simulink model "takeoff23b"  (R2025b)
settings: Solver=ode4  StartTime=0.0  StopTime=150  FixedStep=0.001  RelTol=1e-3
values from neighbouring files (symbols this model uses):
  a0 = 340.294    [basedata.m]    (also in basedata.mat; landing_init.m; landing_plan.mat; landingplan.mat)
  b_ref = 2.0    (= 2)    [basedata.m]    (also in basedata.mat; landing_init.m; landing_plan.mat; landingplan.mat)
  c_gear = [0.8e4, 1.4e4, 1.4e4]    [basedata.m]    (also in basedata.mat = [8000 14000 14000]; landing_init.m; landing_plan.mat = [8000 14000 14000]; landingplan.mat = [8000 14000 14000])
  c_lat = [1.4e4, 2.2e4, 2.2e4]    [basedata.m]    (also in basedata.mat = [14000 22000 22000]; landing_init.m; landing_plan.mat = [14000 22000 22000]; landingplan.mat = [14000 22000 22000])
  c_ref = 0.9    [basedata.m]    (also in basedata.mat; landing_init.m; landing_plan.mat; landingplan.mat)
  c_roll = [0.020, 0.018, 0.018]    [basedata.m]    (also in basedata.mat = [0.02 0.018 0.018]; landing_init.m; landing_plan.mat = [0.02 0.018 0.018]; landingplan.mat = [0.02 0.018 0.018])
  CD0 = 0.045    [basedata.m]    (also in basedata.mat; canshujisuan.m; landing_init.m; landing_plan.mat)
  CL0 = 0.083    [basedata.m]    (also in basedata.mat; landing_init.m; landing_plan.mat; landing_trajectory.m)
  CLa = 3.80    (= 3.8)    [basedata.m]    (also in basedata.mat; canshujisuan.m = 2.5; landing_init.m; landing_plan.mat)
  Clb = -0.08    [basedata.m]    (also in basedata.mat; landing_init.m; landing_plan.mat; landingplan.mat)
  Clda = -0.20    (= -0.2)    [basedata.m]    (also in basedata.mat; landing_init.m; landing_plan.mat; landingplan.mat)
  CLde = 0.28    [basedata.m]    (also in basedata.mat; landing_init.m; landing_plan.mat; landingplan.mat)
  Clp = -0.70    (= -0.7)    [basedata.m]    (also in basedata.mat; landing_init.m; landing_plan.mat; landingplan.mat)
  CLq = 4.50    (= 4.5)    [basedata.m]    (also in basedata.mat; canshujisuan.m = 3; landing_init.m; landing_plan.mat)
  Clr = 0.08    [basedata.m]    (also in basedata.mat; landing_init.m; landing_plan.mat; landingplan.mat)
  Cm0 = 0.060    (= 0.06)    [basedata.m]    (also in basedata.mat; landing_init.m; landing_plan.mat; landingplan.mat)
  Cma = -0.80    (= -0.8)    [basedata.m]    (also in basedata.mat; landing_init.m; landing_plan.mat; landingplan.mat)
  Cmde = -0.90    (= -0.9)    [basedata.m]    (also in basedata.mat; landing_init.m; landing_plan.mat; landingplan.mat)
  Cmq = -18.0    (= -18)    [basedata.m]    (also in basedata.mat; landing_init.m; landing_plan.mat; landingplan.mat)
  Cnb = 0.25    [basedata.m]    (also in basedata.mat; landing_init.m; landing_plan.mat; landingplan.mat)
  Cndr = -0.15    [basedata.m]    (also in basedata.mat; landing_init.m; landing_plan.mat; landingplan.mat)
  Cnp = -0.04    [basedata.m]    (also in basedata.mat; landing_init.m; landing_plan.mat; landingplan.mat)
  Cnr = -0.45    [basedata.m]    (also in basedata.mat; landing_init.m; landing_plan.mat; landingplan.mat)
  CSb = -0.70    (= -0.7)    [basedata.m]    (also in basedata.mat; landing_init.m; landing_plan.mat; landingplan.mat)
  CSdr = 0.18    [basedata.m]    (also in basedata.mat; landing_init.m; landing_plan.mat; landingplan.mat)
  CSr = 0.12    [basedata.m]    (also in basedata.mat; landing_init.m; landing_plan.mat; landingplan.mat)
  D = 0.5 * rho0 * V^2 * S_ref * CD_current    [canshujisuan.m]
  D0 = 1400    [basedata.m]    (also in basedata.mat; landing.m; landing_init.m; landing_plan.mat)
  da_max = 25    [basedata.m]    (also in basedata.mat; landing_init.m; landing_plan.mat; landingplan.mat)
  da_min = -da_max    (= -25)    [basedata.m]    (also in basedata.mat; landing_init.m; landing_plan.mat; landingplan.mat)
  de_max = 25    [basedata.m]    (also in basedata.mat; landing_init.m; landing_plan.mat; landingplan.mat)
  de_min = -de_max    (= -25)    [basedata.m]    (also in basedata.mat; landing_init.m; landing_plan.mat; landingplan.mat)
  DH = pi / 180    (= 0.0174532925199)    [basedata.m]    (also in basedata.mat; landing_init.m; landing_plan.mat; landingplan.mat)
  dr_max = 25    [basedata.m]    (also in basedata.mat; landing_init.m; landing_plan.mat; landingplan.mat)
  dr_min = -dr_max    (= -25)    [basedata.m]    (also in basedata.mat; landing_init.m; landing_plan.mat; landingplan.mat)
  g = 9.80665    [basedata.m]    (also in basedata.mat; canshujisuan.m; landing_init.m; landing_plan.mat)
  gamma1 = -0.125844364415    [basedata.mat]    (also in landing_trajectory.m = asin((T_idle - D_app) / (m*g)); landingplan.mat)
  gamma2 = -0.0261780104712    [basedata.mat]    (also in landing_trajectory.m; landingplan.mat)
  ground_z = 0.0    (= 0)    [basedata.m]    (also in basedata.mat; landing_init.m; landing_plan.mat; landingplan.mat)
  HD = 180 / pi    (= 57.2957795131)    [basedata.m]    (also in basedata.mat; landing_init.m; landing_plan.mat; landingplan.mat)
  I = [ Ixx, -Ixy, -Ixz ... (first row only)    [basedata.m]    (also in basedata.mat = [120  0  0; 0  480  0; 0  0  520]; landing_init.m; landing_plan.mat = [120  0  0; 0  480  0; 0  0  520]; landingplan.mat = [120  0  0; 0  480  0; 0  0  520])
  K = 0.12    [basedata.m]    (also in basedata.mat; canshujisuan.m = 0.08; landing_init.m; landing_plan.mat)
  K_alpha = 7.5375    [basedata.mat]    (also in control_design.m = (((wd_pitch^2)-a24))/(2*kesi_pitch*wd_pitch); control_design.mat; controller.m = 5; landingplan.mat)
  k_gear = [1.0e5, 3.0e5, 3.0e5]    [basedata.m]    (also in basedata.mat = [100000 300000 300000]; landing_init.m; landing_plan.mat = [100000 300000 300000]; landingplan.mat = [100000 300000 300000])
  Kn_pitch = -0.120095403309    [basedata.mat]    (also in control_design.m = -(2.2*g*(wd_pitch)^2)/(Tr*(((wd_pitch)^2)-a24)*V_control*a34; control_design.mat; controller.m = (2.2*wd^2*g)/(Tr*(wd^2-a24)*V_test*a34); landingplan.mat)
  Kw_pitch = -0.483749055178    [basedata.mat]    (also in control_design.m = -2*kesi_pitch*wd_pitch/a25; control_design.mat; controller.m = -(2*zeta*wd) / a25; landingplan.mat)
  m = 600.0    (= 600)    [basedata.m]    (also in basedata.mat; canshujisuan.m; landing_init.m; landing_plan.mat)
  mu_brake = [0.0, 0.55, 0.55]    [basedata.m]    (also in basedata.mat = [0 0.55 0.55]; landing_init.m; landing_plan.mat = [0 0.55 0.55]; landingplan.mat = [0 0.55 0.55])
  phi0 = 0.0    (= 0)    [landing.m]    (also in landing_init.m; landing_init.mat; landing_plan.mat; landingplan.mat)
  psi0 = 0.0    (= 0)    [landing.m]    (also in landing_init.m; landing_init.mat; landing_plan.mat; landingplan.mat)
  r_left_b = r_gear_b(:,2)    [basedata.m]    (also in basedata.mat = [-0.333333333333 -0.8 0.65]; landing_init.m; landing_plan.mat = [-0.333333333333 -0.8 0.65]; landingplan.mat = [-0.333333333333 -0.8 0.65])
  r_nose_b = r_gear_b(:,1)    [basedata.m]    (also in basedata.mat = [2 0 0.65]; landing_init.m; landing_plan.mat = [2 0 0.65]; landingplan.mat = [2 0 0.65])
  r_right_b = r_gear_b(:,3)    [basedata.m]    (also in basedata.mat = [-0.333333333333 0.8 0.65]; landing_init.m; landing_plan.mat = [-0.333333333333 0.8 0.65]; landingplan.mat = [-0.333333333333 0.8 0.65])
  rho0 = 1.225    [basedata.m]    (also in basedata.mat; canshujisuan.m; landing_init.m; landing_plan.mat)
  S_ref = 1.2    [basedata.m]    (also in basedata.mat; canshujisuan.m; landing_init.m; landing_plan.mat)
  theta0 = 0.0    (= 0)    [landing.m]    (also in landing_init.m; landing_init.mat = 0.0523598775598; landing_plan.mat = 0.0523560209424; landingplan.mat)
  u0_b = 128.0    (= 128)    [landing.m]    (also in landing_init.m; landing_init.mat = 100; landing_plan.mat; landingplan.mat)
  v0_b = 0.0    (= 0)    [landing.m]    (also in landing_init.m; landing_init.mat; landing_plan.mat; landingplan.mat)
  v_eps = 0.20    (= 0.2)    [basedata.m]    (also in basedata.mat; landing_init.m; landing_plan.mat; landingplan.mat)
  V_min = 3    [landing.m]    (also in landing_init.m; landing_plan.mat; landingplan.mat; plan.m = 1)
  w0_b = 0.0    (= 0)    [landing.m]    (also in landing_init.m; landing_init.mat; landing_plan.mat; landingplan.mat)
  wheel_radius = 0.18    [basedata.m]    (also in basedata.mat; landing_init.m; landing_plan.mat; landingplan.mat)
  WOW_on = 0.000    (= 0)    [basedata.m]    (also in basedata.mat; landing_init.m; landing_plan.mat; landingplan.mat)
  Xg0 = -12000.0    (= -12000)    [landing.m]    (also in landing_init.m; landing_init.mat = -8000; landing_plan.mat; landingplan.mat)
  Yg0 = 0.0    (= 0)    [landing.m]    (also in landing_init.m; landing_init.mat; landing_plan.mat; landingplan.mat)
  Zg0 = ground_z - wheel_radius - r_gear_b(3,1) + static_deflection    [basedata.m]    (also in basedata.mat = -0.8215943; landing.m = -1000; landing_init.m = -1000; landing_init.mat = -350)
undefined symbols (not defined in the file or in its folder): I_xz, I_yz, Ix_Iy, Iy_Iz, Iz_Ix
libraries: simulink x58, matrix_library x19
(part 4 of 4)

== matlab function takeoff23b/6DOF-MODEL/动力学/Subsystem3/MATLAB Function ==
  data: phi input; R_bg output; theta input; psi input
function R_bg = ground2body(phi, theta, psi)
T1 = [cos(psi), sin(psi), 0;
     -sin(psi), cos(psi), 0;
      0, 0, 1];
T2 = [cos(theta), 0, -sin(theta);
       0, 1, 0;
      sin(theta), 0, cos(theta)];
T3 = [1, 0, 0;
      0, cos(phi), sin(phi);
      0, -sin(phi), cos(phi)];
R_bg = T3 * T2 * T1;

== matlab function takeoff23b/6DOF-MODEL/动力学/dynamics EQ/MATLAB Function ==
  data: alpha input; R_bwind output; beta input
function R_bwind = wind2body(alpha, beta)
T1 = [cos(alpha), 0, sin(alpha);
       0, 1, 0;
       -sin(alpha), 0, cos(alpha)];
T2 = [cos(beta), sin(beta), 0;
       -sin(beta), cos(beta), 0;
       0, 0, 1];
R_wind_b = T2*T1;
R_bwind = R_wind_b';

== matlab function takeoff23b/controller1/4_Power&V_Ctrl/MATLAB Function ==
  data: Vel_g input; dv_err output; axyz input
function dv_err = dv_cal(Vel_g,axyz)
%#codegen

% k_theta = Att_g(1)*pi/180;
% psi = Att_g(2)*pi/180;
% gama = Att_g(3)*pi/180;
% 
% Cg_b = Mx(gama)*Mz(k_theta)*My(psi);
% Cb_g = Cg_b';
vx = Vel_g(1);
vy = Vel_g(2);
vz = Vel_g(3);

ax = axyz(1);
ay = axyz(2);
az = axyz(3);

dv_err = (vx*ax + vy*ay + vz*az)/sqrt(vx^2 + vy^2 + vz^2);
% dv_err = (vx*ax + vz*az)/sqrt(vx^2 + vz^2);
if isnan(dv_err) == 1 
    dv_err = 0;
end

== matlab function takeoff23b/6DOF-MODEL/动力学/dynamics EQ/MATLAB Function1 ==
  data: phi input; R_bg output; theta input; psi input
function R_bg = ground2body(phi, theta, psi)
T1 = [cos(psi), sin(psi), 0;
     -sin(psi), cos(psi), 0;
      0, 0, 1];
T2 = [cos(theta), 0, -sin(theta);
       0, 1, 0;
      sin(theta), 0, cos(theta)];
T3 = [1, 0, 0;
      0, cos(phi), sin(phi);
      0, -sin(phi), cos(phi)];
R_bg = T3 * T2 * T1;

== matlab function takeoff23b/6DOF-MODEL/动力学/height/MATLAB Function ==
  data: phi input; R_bg output; theta input; psi input
function R_bg = ground2body(phi, theta, psi)
T1 = [cos(psi), sin(psi), 0;
     -sin(psi), cos(psi), 0;
      0, 0, 1];
T2 = [cos(theta), 0, -sin(theta);
       0, 1, 0;
      sin(theta), 0, cos(theta)];
T3 = [1, 0, 0;
      0, cos(phi), sin(phi);
      0, -sin(phi), cos(phi)];
R_bg = T3 * T2 * T1;

== matlab function takeoff23b/6DOF-MODEL/动力学/rotation EQ/MATLAB Function1 ==
  data: w input; wB_X output
function wB_X = wB_X(w) 
p = w(1);
q = w(2);
r = w(3);
wB_X = [0, -r,  q;...
        r,  0, -p;...
       -q,  p,  0];

== matlab function takeoff23b/6DOF-MODEL/动力学/起落架模型/MATLAB Function ==
  data: phi input; R_bg output; theta input; psi input
function R_bg = ground2body(phi, theta, psi)
T1 = [cos(psi), sin(psi), 0;
     -sin(psi), cos(psi), 0;
      0, 0, 1];
T2 = [cos(theta), 0, -sin(theta);
       0, 1, 0;
      sin(theta), 0, cos(theta)];
T3 = [1, 0, 0;
      0, cos(phi), sin(phi);
      0, -sin(phi), cos(phi)];
R_bg = T3 * T2 * T1;

== matlab function takeoff23b/6DOF-MODEL/动力学/起落架模型/侧向力/Subsystem/MATLAB Function ==
  data: phi input; R_bg output; theta input; psi input
function R_bg = ground2body(phi, theta, psi)
T1 = [cos(psi), sin(psi), 0;
     -sin(psi), cos(psi), 0;
      0, 0, 1];
T2 = [cos(theta), 0, -sin(theta);
       0, 1, 0;
      sin(theta), 0, cos(theta)];
T3 = [1, 0, 0;
      0, cos(phi), sin(phi);
      0, -sin(phi), cos(phi)];
R_bg = T3 * T2 * T1;

== matlab function takeoff23b/6DOF-MODEL/动力学/起落架模型/侧向力/Subsystem/主轮侧向方向向量 ==
  data: Cbg input; eg_lat output; eb_lat input
function eg_lat = project_main_lat(Cbg, eb_lat)

e_z = [0; 0; 1];              % 前-右-下坐标系：Z 轴向下
P_g = eye(3) - e_z*e_z.';     % 投影到地面水平面

eg_lat = P_g * Cbg * eb_lat;

n = norm(eg_lat);
if n > 1e-8
    eg_lat = eg_lat / n;
else
    eg_lat = [0; 1; 0];       % 默认地面右向
end

== matlab function takeoff23b/6DOF-MODEL/动力学/起落架模型/侧向力/Subsystem/前轮侧向向量 ==
  data: Cbg input; eg_lat output; eb_lat input
function eg_lat = project_lat(Cbg, eb_lat)

e_z = [0; 0; 1];              % 前-右-下坐标系：Z 轴向下
P_g = eye(3) - e_z*e_z.';     % 投影到地面水平面

eg_lat = P_g * Cbg * eb_lat;

n = norm(eg_lat);
if n > 1e-8
    eg_lat = eg_lat / n;
else
    eg_lat = [0; 1; 0];       % 默认地面右向
end

== matlab function takeoff23b/6DOF-MODEL/动力学/起落架模型/MATLAB Function1 ==
  data: phi input; R_bg output; theta input; psi input
function R_bg = ground2body(phi, theta, psi)
T1 = [cos(psi), sin(psi), 0;
     -sin(psi), cos(psi), 0;
      0, 0, 1];
T2 = [cos(theta), 0, -sin(theta);
       0, 1, 0;
      sin(theta), 0, cos(theta)];
T3 = [1, 0, 0;
      0, cos(phi), sin(phi);
      0, -sin(phi), cos(phi)];
R_bg = T3 * T2 * T1;

== matlab function takeoff23b/6DOF-MODEL/动力学/起落架模型/三轮在地系下的力/摩擦圆限幅/前轮摩擦圆限幅 ==
  data: N input; F_long_out output; F_long input; F_lat input; F_lat_out output
function [F_long_out,F_lat_out]=Dround_saturation_nose(N,F_long,F_lat)
mu=0.65;
F_ALL=sqrt((F_long)^2+(F_lat)^2);
if(F_ALL<=mu*N)
    F_long_out=F_long;
    F_lat_out=F_lat;
else
    s=mu*N/F_ALL;
    F_long_out=s*F_long;
    F_lat_out=s*F_lat;
end

== matlab function takeoff23b/6DOF-MODEL/动力学/起落架模型/三轮在地系下的力/摩擦圆限幅/主轮摩擦圆限幅左 ==
  data: N input; F_long_out output; F_long input; F_lat input; F_lat_out output
function [F_long_out,F_lat_out]=Dround_saturation_main(N,F_long,F_lat)
mu=0.7;
F_ALL=sqrt((F_long)^2+(F_lat)^2);
if(F_ALL<=mu*N)
    F_long_out=F_long;
    F_lat_out=F_lat;
else
    s=mu*N/F_ALL;
    F_long_out=s*F_long;
    F_lat_out=s*F_lat;
end

== matlab function takeoff23b/6DOF-MODEL/动力学/起落架模型/三轮在地系下的力/摩擦圆限幅/主轮摩擦圆限幅右 ==
  data: N input; F_long_out output; F_long input; F_lat input; F_lat_out output
function [F_long_out,F_lat_out]=Dround_saturation_main(N,F_long,F_lat)
mu=0.7;
F_ALL=sqrt((F_long)^2+(F_lat)^2);
if(F_ALL<=mu*N)
    F_long_out=F_long;
    F_lat_out=F_lat;
else
    s=mu*N/F_ALL;
    F_long_out=s*F_long;
    F_lat_out=s*F_lat;
end

== matlab function takeoff23b/Guidance/3_空中制导/高度切换/MATLAB Function ==
  data: X_pos input; Hcmd output
function Hcmd = round_hcmd(X_pos)

X_B = -4048.3;
X_C = -3253.6;
X_R = -3044.2;
H_R = 8069.4;
R = 8000;

if X_pos >= X_B && X_pos <= X_C
    rad = R^2 - (X_pos - X_R)^2;
    Hcmd = H_R - sqrt(max(rad, 0));
else
    Hcmd = 0;
end

== matlab function takeoff23b/6DOF-MODEL/动力学/起落架模型/法向支反力/MATLAB Function ==
  data: phi input; R_bg output; theta input; psi input
function R_bg = ground2body(phi, theta, psi)
T1 = [cos(psi), sin(psi), 0;
     -sin(psi), cos(psi), 0;
      0, 0, 1];
T2 = [cos(theta), 0, -sin(theta);
       0, 1, 0;
      sin(theta), 0, cos(theta)];
T3 = [1, 0, 0;
      0, cos(phi), sin(phi);
      0, -sin(phi), cos(phi)];
R_bg = T3 * T2 * T1;

== matlab function takeoff23b/6DOF-MODEL/动力学/height/MATLAB Function1 ==
  data: phi input; R_bg output; theta input; psi input
function R_bg = ground2body(phi, theta, psi)
T1 = [cos(psi), sin(psi), 0;
     -sin(psi), cos(psi), 0;
      0, 0, 1];
T2 = [cos(theta), 0, -sin(theta);
       0, 1, 0;
      sin(theta), 0, cos(theta)];
T3 = [1, 0, 0;
      0, cos(phi), sin(phi);
      0, -sin(phi), cos(phi)];
R_bg = T3 * T2 * T1;

== stateflow chart takeoff23b/Flight Phase Manager/Phase Logic ==
  state Takeoff_Mode
    state Ground_Roll
      en: Flight_Phase = 1;
    state Rotation
      en: Flight_Phase = 2;
    state Liftoff
      en: Flight_Phase = 3;
    state Initial_Climb
      en: Flight_Phase = 4;
    state Climb_Complete
      en: Flight_Phase = 5;
    (default) -> Ground_Roll
    Ground_Roll -> Rotation : [reach_VR == true]
    Rotation -> Liftoff : [airborne == true]
    Liftoff -> Initial_Climb : [safe_climb == true]
    Initial_Climb -> Climb_Complete : [h_AGL  >= 800.0]
  state Landing_Mode
    state Glideslope_Capture
      en: Flight_Phase = 7;
    state Glideslope_Track
      en: Flight_Phase = 8;
    state Approach_Turn
      en: Flight_Phase = 6;
    state Roll_out
      en: Flight_Phase = 11;
    state Touchdown
      en: Flight_Phase = 10;
    state RoundFlare
      en: Flight_Phase = 9;
    (default) -> Approach_Turn
    Approach_Turn -> Glideslope_Capture : [localizer_captured == true]
    Glideslope_Capture -> Glideslope_Track : [glideslope_captured == true]
    Glideslope_Track -> RoundFlare : [In_round == true]
    Touchdown -> Roll_out : [nose_on_ground == true && V_runway < 35.0]
    RoundFlare -> Touchdown : [Slight_decline == true]
  (junction 38) -> Takeoff_Mode [order 1] : [Task_Mode == 1]{Flight_Phase = 0;}
  (default) -> (junction 38)
  (junction 38) -> Landing_Mode [order 2] : {Flight_Phase = 0;}
  data: h_AGL input size=1; V_runway input size=1; h_dot input; nose_on_ground input size=1; main_on_ground input size=1; airborne input size=1; reach_VR input size=1; safe_climb input size=1; localizer_captured input size=1; glideslope_captured input size=1; flare_entry input size=1; stop_condition input size=1; Task_Mode input size=1; Flight_Phase output uint8 size=1 =0; In_round input; Slight_decline input

== matlab function takeoff23b/6DOF-MODEL/动力学/起落架模型/纵向力/Subsystem/MATLAB Function ==
  data: phi input; R_bg output; theta input; psi input
function R_bg = ground2body(phi, theta, psi)
T1 = [cos(psi), sin(psi), 0;
     -sin(psi), cos(psi), 0;
      0, 0, 1];
T2 = [cos(theta), 0, -sin(theta);
       0, 1, 0;
      sin(theta), 0, cos(theta)];
T3 = [1, 0, 0;
      0, cos(phi), sin(phi);
      0, -sin(phi), cos(phi)];
R_bg = T3 * T2 * T1;

== matlab function takeoff23b/6DOF-MODEL/动力学/起落架模型/纵向力/Subsystem/主轮滚动方向向量 ==
  data: Cbg input; eg_long output; eb_long input
function eg_long = project_long(Cbg, eb_long)

e_z = [0; 0; 1];              % 前-右-下坐标系：Z 轴向下
P_g = eye(3) - e_z*e_z.';     % 投影到地面水平面

eg_long = P_g * Cbg * eb_long;

n = norm(eg_long);
if n > 1e-8
    eg_long = eg_long / n;
else
    eg_long = [1; 0; 0];
end

== matlab function takeoff23b/6DOF-MODEL/动力学/起落架模型/纵向力/Subsystem/前轮滚动方向向量 ==
  data: Cbg input; eg_long output; eb_long input
function eg_long = project_long(Cbg, eb_long)

e_z = [0; 0; 1];              % 前-右-下坐标系中，Z 轴为下
P_g = eye(3) - e_z*e_z.';     % 投影到地面水平面

eg_long = P_g * Cbg * eb_long;

n = norm(eg_long);
if n > 1e-8
    eg_long = eg_long / n;
else
    eg_long = [1; 0; 0];
end

== matlab function takeoff23b/6DOF-MODEL/动力学/起落架模型/起落架三轮质心在地系下位置/MATLAB Function ==
  data: phi input; R_bg output; theta input; psi input
function R_bg = ground2body(phi, theta, psi)
T1 = [cos(psi), sin(psi), 0;
     -sin(psi), cos(psi), 0;
      0, 0, 1];
T2 = [cos(theta), 0, -sin(theta);
       0, 1, 0;
      sin(theta), 0, cos(theta)];
T3 = [1, 0, 0;
      0, cos(phi), sin(phi);
      0, -sin(phi), cos(phi)];
R_bg = T3 * T2 * T1;

== matlab function takeoff23b/controller1/4_Power&V_Ctrl/MATLAB Function1 ==
  settings: updateMethod=DISCRETE  sampleTime=0.001
  data: phase input; throttle_out output; throttle_direct input; throttle_speed input; t input; T_blend input; lambda output
function [throttle_out, lambda] = phase4_to_5_blend(phase, throttle_direct, throttle_speed, t, T_blend)
%#codegen
persistent t_enter5 last_phase throttle_start last_out

if isempty(t_enter5)
    t_enter5 = -1.0;
    last_phase = phase;
    throttle_start = throttle_direct;
    last_out = throttle_direct;
end

if T_blend <= 0
    T_blend = 3.0;
end

if phase < 5
    lambda = 0.0;
    throttle_out = throttle_direct;
    t_enter5 = -1.0;
    throttle_start = throttle_direct;
else
    if last_phase < 5 || t_enter5 < 0
        t_enter5 = t;
        throttle_start = last_out;
    end

    tau = (t - t_enter5) / T_blend;

    if tau < 0
        tau = 0;
    elseif tau > 1
        tau = 1;
    end

    lambda = tau * tau * (3.0 - 2.0 * tau);

    throttle_out = (1.0 - lambda) * throttle_start + lambda * throttle_speed;
end

if throttle_out > 1.0
    throttle_out = 1.0;
elseif throttle_out < 0.0
    throttle_out = 0.0;
end

last_phase = phase;
last_out = throttle_out;
